simulink model "closedloop_leadlag"  (R2020b)
settings: Solver=VariableStepAuto  StartTime=0.0  StopTime=10.0  FixedStep=0.00002  RelTol=1e-3
undefined symbols (not defined in the file): B_e, J_e, K_a, K_e, K_t, mu_k, sat, T, t_start
libraries: cstblocks x3
settings Model: Creator=jasper  LastModifiedBy=jasper

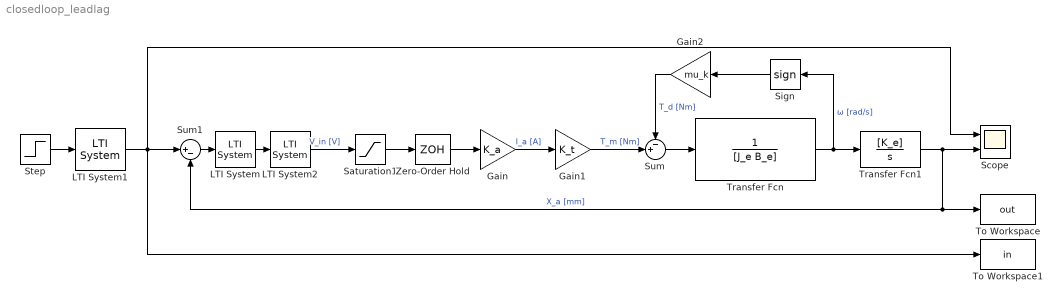
== system closedloop_leadlag ==
  Gain : Gain  Gain=K_a
  Gain1 : Gain  Gain=K_t
  Gain2 : Gain  Gain=mu_k
  LTI System : cstblocks/LTI System  sys=C_comp  IC=[]
  LTI System1 : cstblocks/LTI System  sys=ref_in  IC=[]
  LTI System2 : cstblocks/LTI System  sys=int_act  IC=[]
  Saturation1 : Saturate  UpperLimit=sat  LowerLimit=-sat  ZeroCross=off
  Scope : Scope  NumInputPorts=2
  Sign : Signum  ZeroCross=off
  Step : Step  Time=t_start  SampleTime=0
  Sum : Sum  Inputs=-+|
  Sum1 : Sum  Inputs=|+-
  To Workspace : ToWorkspace  VariableName=out  SaveFormat=Timeseries  SampleTime=-1
  To Workspace1 : ToWorkspace  VariableName=in  SaveFormat=Timeseries  SampleTime=-1
  Transfer Fcn : TransferFcn  Denominator=[J_e B_e]
  Transfer Fcn1 : TransferFcn  Numerator=[K_e]  Denominator=[1 0]
  Zero-Order Hold : ZeroOrderHold  SampleTime=T
  wires:
  Saturation1/1 -> Zero-Order Hold/1
  Zero-Order Hold/1 -> Gain/1
  Gain/1 -> Gain1/1  "I_a [A]"
  Gain1/1 -> Sum/2  "T_m [Nm]"
  Sum/1 -> Transfer Fcn/1
  Sign/1 -> Gain2/1
  Gain2/1 -> Sum/1  "T_d [Nm]"
  Transfer Fcn/1 -> Transfer Fcn1/1, Sign/1  "ω [rad/s]"
  Transfer Fcn1/1 -> Scope/2, To Workspace/1, Sum1/2  "X_a [mm]"
  Sum1/1 -> LTI System/1
  LTI System1/1 -> Scope/1, To Workspace1/1, Sum1/1
  Step/1 -> LTI System1/1
  LTI System/1 -> LTI System2/1
  LTI System2/1 -> Saturation1/1  "V_in [V]"
